simulink model "PID_Loop_2023a"  (R2025a)
settings: Solver=FixedStepAuto  StartTime=0.0  StopTime=tspan  FixedStep=dt  RelTol=1e-3
model workspace (MAT data in the model file):
  Drag_Constants = 1
  mass = [5.51 5.51 5.51 1 1 1]
  mass_6a = [5 5 5 1 1 1]
undefined symbols (not defined in the file): bin_loc, do_bouyancy_flag, do_control_force_flag, do_drag_flag, do_gravity_flag, drag_wrench, dt, Dt, dt_controller, dt_filter, dt_imu, dt_plotting, fractalcoef, g, H, IMU, inverse_wrench, max_pitch_torque, max_roll_torque, max_xyz_force, max_yaw_torque, P, pool_depth, Q, R, states_desired, v0_e, volume, volume_center, w0, water_density, waypoints, wrench, x0_e
libraries: slpidlib x4, aerolibobsolete x1, mspfiltlib x1, mspsensorlib x1
(part 2 of 2)

== matlab function PID_Loop_2023a/Plant/Thruster Forces/PWM to Motor Forces ==
  data: thruster_pwms input; forces_N output
function forces_N  = fcn(thruster_pwms)
    %{
        This function  uses a polynomial fit to the pwm vs thrust curve 
        for the T200 Thrusters to calculate the 8 thruster force vectors.
    %}
    %preallocate
    forces_N = zeros(size(thruster_pwms)); 
    
    
    % First condition: 1100 <= x < 1460
    index_array = (thruster_pwms >= 1100 & thruster_pwms < 1460);

    
    forces_N(index_array) =  (-1.76709811615214e-07) * thruster_pwms(index_array).^3 ...
                 + (0.000566300482093069) * thruster_pwms(index_array).^2 ...
                 + (-0.478920592563405) * thruster_pwms(index_array) ...
                 + 41.55273858905;
    
    % Second condition: 1460 <= x <= 1540
    index_array = (thruster_pwms >= 1460 & thruster_pwms <= 1540);
    forces_N(index_array) = 0;
    
    % Third condition: 1540 < x <= 1900
    index_array = (thruster_pwms > 1540 & thruster_pwms <= 1900);
    forces_N(index_array) = (-1.81933850672702e-07) * thruster_pwms(index_array).^3 ...
                 + (0.00109777888824906) * thruster_pwms(index_array).^2 ...
                 + (-2.03121269418349) * thruster_pwms(index_array) ...
                 + (1189.65910925401);
    
    % Handle out-of-range values
    if any(isnan(forces_N))
        error('Some values in x_array are out of the valid range [1100..1900].');
    end

    
end

== matlab function PID_Loop_2023a/Sensors/eul2rotm ==
  data: Eulers input; DCMbe output
function DCMbe = fcn(Eulers)

DCMbe = eul2rotm([Eulers(3), Eulers(2), Eulers(1)]);

== matlab function PID_Loop_2023a/Controller/Thruster Forces to PWM ==
  data: thruster_force_cmd input; pwm_cmd output
function pwm_cmd = fcn(thruster_force_cmd)

pwm_cmd = zeros(8,1);
%uses a curve fit for thrust to pwm from the t200 thruster data sheet

for i=1:length(pwm_cmd)
    x = thruster_force_cmd(i);
    y = 0;

    if(x>0)
        y = round(0.00231011300235566*x^3 + -0.229204832763592*x^2 + 13.7272237851422*x + 1536.34500151024);
    elseif(x<0)
        y = round(0.00475737746846442*x^3 + 0.360062809963915*x^2 + 17.2034080439155*x + 1463.91061014397);
    else
        y = 1500;
    end

    %saturation
    if(y > 1900)
        y = 1900;
    end
    if (y < 1100)
        y = 1100;
    end

    pwm_cmd(i) = y;

end

== matlab function PID_Loop_2023a/Plant/Gravity and Hydrostatics/Bouyant Force ==
  data: DCMbe input; buoyant_force output; g parameter; water_density parameter; volume parameter; volume_center parameter
function buoyant_force = buoyant_force(DCMbe, g, water_density, volume, volume_center)

    % Ensure d is a column vector
    volume_center = volume_center(:);

    % Buoyant force vector in world frame
    b_vector = [0; 0; water_density * -g * volume];

    % Rotate buoyant force to object's frame
    buoyant_force_body = DCMbe * b_vector;

    % Compute torque using cross product τ = d × F_buoyancy
    % (MATLAB cross function works for column vectors)
    torque = cross(volume_center, buoyant_force_body);

    % Combine force and torque into a single output vector
    buoyant_force = [buoyant_force_body; torque];
end

== matlab function PID_Loop_2023a/Plant/Gravity and Hydrostatics/Weight ==
  data: DCMbe input; weight_force output; g parameter; P parameter; g_b output
function [weight_force,g_b] = weight_force(DCMbe, g, P)
    m = P.m;

    % Gravity force vector in world frame (downward)
    g_vector = [0; 0; m * g];
    
    % Linear Force
    lin = DCMbe * g_vector;
    g_b = DCMbe * [0;0;g];
    % Rotational force
    rot = [0;0;0];
    % Transform gravity force to rotated frame
    weight_force = [lin; rot];
end

== matlab function PID_Loop_2023a/Waypoint Follower/Desired State Generator ==
  data: current_waypoint output; waypoints input; desired_states output; states_des input; current_waypoint_index output; current_waypoint_index input; intermediate_waypoint input; tol parameter; intermediate_waypoint output
function [current_waypoint,desired_states,current_waypoint_index,intermediate_waypoint]= fcn(waypoints,states_des,current_waypoint_index,intermediate_waypoint,tol)

%The initial value of the current_waypoint_index is 1, as set in the data
%store memory block.
x_e = states_des(1:3);

% check the next waypoint in the list
current_waypoint = waypoints(:,current_waypoint_index);

%get the length of the waypoint list
[~, N_wp] = size(waypoints);
% get the position vector to the current waypoint
r_b2wp_e = current_waypoint - x_e;
%get the range to the current waypoint
R_wp = norm(r_b2wp_e);

% get the range to the current intermediate waypoint
r_b2iwp_e = intermediate_waypoint - x_e;
R_int_wp = norm(r_b2iwp_e);

% if the range to the intermediate waypoint is smaller than the tolerance
if(R_wp <= tol)
    %if there is another waypoint on the list, switch the current waypoint
    %to that
    if(current_waypoint_index < N_wp)
        current_waypoint_index = current_waypoint_index + 1; %update wp index
        current_waypoint = waypoints(:,current_waypoint_index); %update wp
    else
        %keep using the current waypoint without changing it
        current_waypoint_index = N_wp;
        current_waypoint = current_waypoint; 
    end
    %recalculate the range
    r_b2wp_e = current_waypoint - x_e;
    R_wp = norm(r_b2wp_e);
end

%if the range to the waypoint and intermediate waypoint is larger than 1
if(R_wp > 1 && R_int_wp > 1)
    %create an intermediate waypoint
    intermediate_waypoint = x_e + r_b2wp_e/R_wp;
    r_b2iwp_e = intermediate_waypoint - x_e;
    R_int_wp = norm(r_b2iwp_e);

%if the range to the waypoint is greater than 1 but the vehicle is close
%the intermediate waypoint 
elseif(R_wp > 1 && R_int_wp <= 1 && R_int_wp > tol)
    %keep using the intermediate waypoint
    intermediate_waypoint = intermediate_waypoint;

%if the vehicle is far from the current waypoint but has reached the
%intermediate waypoint
elseif(R_wp > 1 && R_int_wp <= tol)
    %generate a new intermediate waypoint
    intermediate_waypoint = x_e + r_b2wp_e/R_wp;

%if the vehicle is close to the final waypoint, make the intermediate
%waypoint the final waypoint
elseif(R_wp <= 1)
    intermediate_waypoint = current_waypoint;

else
    %this shouldn't be reached, but here just in case
    intermediate_waypoint = current_waypoint;
end

%bearing angle
E = states_des(4:6); %unpack the euler angles
DCMbe = eul2rotm(E'); %calculate the rotation matrix
r_b2iwp_b = DCMbe*r_b2iwp_e; %calculate the bearing vector in the body frame
%xy_r_b2iwp_b = [r_b2iwp_b(1); r_b2iwp_b(2); 0]; %project onto xy plane

%to do: figure this out
yaw = atan2(r_b2iwp_b(1),r_b2iwp_b(2));

%put on interval -pi to pi
if (yaw > pi)
    yaw = yaw - 2*pi;
end

desired_states = [intermediate_waypoint;[0 0 yaw]'];

end

== matlab function PID_Loop_2023a/Attitude EKF/Euler EKF ==
  data: phi_meas input; theta_meas input; phi_hat output; w_meas input; xhat_prior input; P_prior input; theta_hat output; psi_hat output; dt parameter; H parameter; x output; P output; Q parameter; R parameter
function [phi_hat, theta_hat, psi_hat, x, P] = fcn(phi_meas,theta_meas,w_meas,xhat_prior,P_prior,dt, H, Q, R)

%Inputs: 
%   z = [phi_meas, theta_meas]', the measured euler angles
%   w = [p q r]' the measured angular rates
%   dt = timestep

%changed variable names to match source material
z = [phi_meas, theta_meas]';
x = xhat_prior;
rates = w_meas;
P = P_prior;

A = Ajacob(x, rates, dt); %get state transition matrix from linearization

%Predict
xp = fx(x, rates, dt); %use state transition function to get a priori update of states
Pp = A*P*A' + Q; %compute a priori error covariance matrix

K = Pp*H'*inv(H*Pp*H' + R); %compute kalman gain

%Correct using measurements
x = xp + K*(z - H*xp);
P = Pp - K*H*Pp;

%use built in matlab functions to make sure euler angles are in the correct
%domain
eul = [x(1) x(2) x(3)];
rotmZXY = eul2rotm(eul);
eul = rotm2eul(rotmZXY);

%outputs
phi_hat = eul(1);
theta_hat = eul(2);
psi_hat = eul(3);
x = [phi_hat;theta_hat;psi_hat];



%state transition function
function xp = fx(xhat,rates,dt)
    phi = xhat(1);
    theta = xhat(2);

    p = rates(1);
    q = rates(2);
    r = rates(3);

    xdot = zeros(3,1);

    %euler angle kinematics
    xdot(1) = p + q*sin(phi)*tan(theta) + r*cos(phi)*tan(theta);
    xdot(2) = q*cos(phi) - r*sin(phi);
    xdot(3) = q*sin(phi)*sec(theta) + r*cos(phi)*sec(theta);

    xp = xhat + xdot*dt;

end

%jacobian function
function A = Ajacob(xhat, rates, dt)
    A = zeros(3,3);

    phi = xhat(1);
    theta = xhat(2);

    p = rates(1);
    q = rates(2);
    r = rates(3);

    A(1,1) = q*cos(phi)*tan(theta) - r*sin(phi)*tan(theta);
    A(1,2) = q*sin(phi)*sec(theta)^2 - r*cos(phi)*sec(theta)^2;
    A(1,3) = 0;

    A(2,1) = -q*sin(phi) - r*cos(phi);
    A(2,2) = 0;
    A(2,3) = 0;

    A(3,1) = q*cos(phi)*sec(theta) - r*sin(phi)*sec(theta);
    A(3,2) = q*sin(phi)*sec(theta)*tan(theta) + r*cos(phi)*sec(theta)*tan(theta);
    A(3,3) = 0;

    A = eye(3) + A*dt;
end
end
